simulink model "chap7_3sim"  (Simulink 3.00)
settings: Solver=ode45  StartTime=0.0  StopTime=50  RelTol=1e-3
settings Model: LastModifiedBy=liu

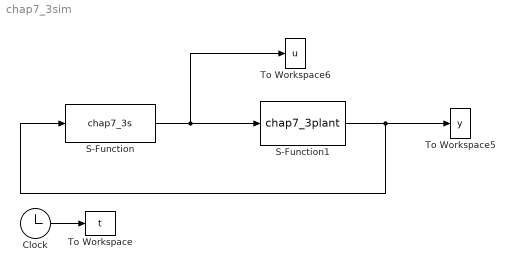
== system chap7_3sim ==
  Clock : Clock
  S-Function : S-Function  FunctionName=chap7_3s  PortCounts=[]  SFunctionModules=''
  S-Function1 : S-Function  FunctionName=chap7_3plant  PortCounts=[]  SFunctionModules=''
  To Workspace : ToWorkspace  VariableName=t  SampleTime=-1  SaveFormat=Matrix
  To Workspace5 : ToWorkspace  VariableName=y  SampleTime=-1  SaveFormat=Matrix
  To Workspace6 : ToWorkspace  VariableName=u  SampleTime=-1  SaveFormat=Matrix
  wires:
  S-Function1/1 -> S-Function/1, To Workspace5/1
  S-Function/1 -> S-Function1/1, To Workspace6/1
  Clock/1 -> To Workspace/1
